simulink model "modeleAncien"  (R2018a)
settings: Solver=VariableStepAuto  StartTime=0.0  StopTime=10.0  RelTol=1e-3
values from neighbouring files (symbols this model uses):
  a = 0.4    [model.m]
  A = [   cos(psy),  -sin(psy)*cos(phi),     0,  0 ... (first row only)    [init.m]    (also in model.m = [   -d1/m,  0,      0)
  B = [   mvr ... (first row only)    [init.m]    (also in model.m = [0, 0, 0)
settings Model: Creator=Maxence  LastModifiedBy=Maxence

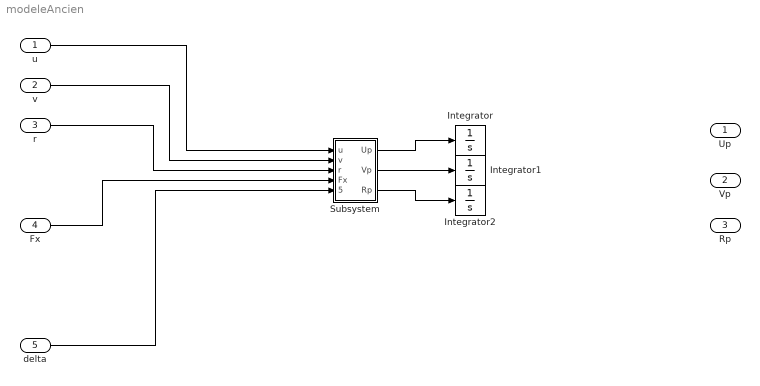
== system modeleAncien ==
  "u " : Inport
  "v " : Inport  Port=2
  r : Inport  Port=3
  Fx : Inport  Port=4
  "delta " : Inport  Port=5
  Integrator : Integrator
  Integrator1 : Integrator
  Integrator2 : Integrator
  Subsystem : Subsystem
  Up : Outport
  "Vp " : Outport  Port=2
  "Rp " : Outport  Port=3
  wires:
  "u "/1 -> Subsystem/1("u ")
  "v "/1 -> Subsystem/2("v ")
  r/1 -> Subsystem/3(r)
  Fx/1 -> Subsystem/4(Fx)
  "delta "/1 -> Subsystem/5("delta ")
  Subsystem/2("Vp ") -> Integrator1/1
  Subsystem/1(Up) -> Integrator/1
  Subsystem/3("Rp ") -> Integrator2/1

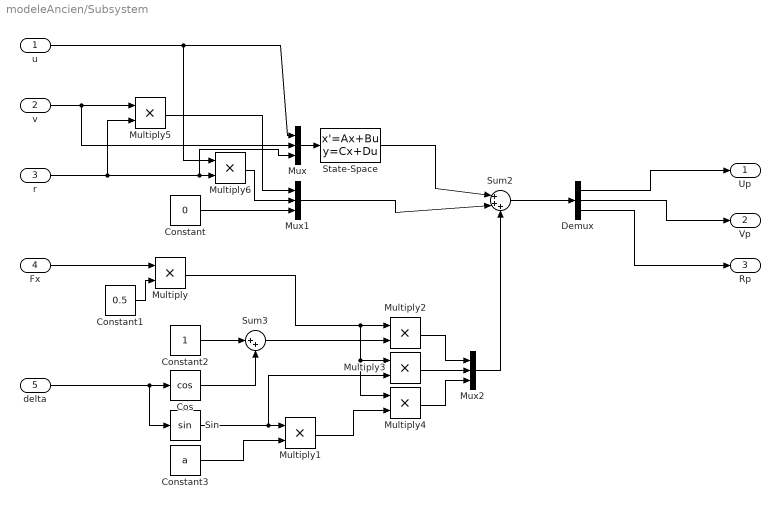
== system modeleAncien/Subsystem ==
  "u " : Inport
  "v " : Inport  Port=2
  r : Inport  Port=3
  Fx : Inport  Port=4
  "delta " : Inport  Port=5
  Constant : Constant  Value=0
  Constant1 : Constant  Value=0.5
  Constant2 : Constant
  Constant3 : Constant  Value=a
  Cos : Trigonometry  Operator=cos
  Demux : Demux  Outputs=3
  Multiply{,1..6} (7 alike) : Product
  Mux : Mux  Inputs=3
  Mux1 : Mux  Inputs=3
  Mux2 : Mux  Inputs=3
  Sin : Trigonometry
  State-Space : StateSpace  A=A  B=B  C=B  D=B  InitialCondition=0
  Sum2 : Sum  Inputs=|+++
  Sum3 : Sum  Inputs=|++
  Up : Outport
  "Vp " : Outport  Port=2
  "Rp " : Outport  Port=3
  wires:
  "u "/1 -> Multiply6/1, Mux/1
  Constant1/1 -> Multiply/2
  Constant/1 -> Mux1/3
  "v "/1 -> Multiply5/1, Mux/2
  Demux/3 -> "Rp "/1
  Multiply5/1 -> Mux1/1
  Sin/1 -> Multiply3/2, Multiply1/1
  "delta "/1 -> Sin/1, Cos/1
  Demux/2 -> "Vp "/1
  Mux/1 -> State-Space/1
  State-Space/1 -> Sum2/1
  Multiply3/1 -> Mux2/2
  r/1 -> Mux/3, Multiply6/2, Multiply5/2
  Mux1/1 -> Sum2/2
  Cos/1 -> Sum3/2
  Sum2/1 -> Demux/1
  Multiply4/1 -> Mux2/3
  Mux2/1 -> Sum2/3
  Demux/1 -> Up/1
  Sum3/1 -> Multiply2/2
  Constant3/1 -> Multiply1/2
  Multiply/1 -> Multiply4/1, Multiply3/1, Multiply2/1
  Constant2/1 -> Sum3/1
  Multiply2/1 -> Mux2/1
  Multiply1/1 -> Multiply4/2
  Fx/1 -> Multiply/1
  Multiply6/1 -> Mux1/2
